simulink model "SR26_2024a"  (R2024a)
settings: Solver=FixedStepDiscrete  StartTime=0.0  StopTime=10.0  FixedStep=0.01  RelTol=1e-3  EnableMultiTasking=on
PreLoadFcn:
  | try, model_open; catch, disp('Error occurred while executing model pre-load callback: model_open.m'); disp('Please assure that the MATLAB working directory is set to the model directory before opening.'); end
InitFcn:
  | try, model_open; catch, end
values from neighbouring files (symbols this model uses):
  dt = 10.0    [SR26.sldd]
undefined symbols (not defined in the file or in its folder): GCM, raptor_get_safe_string, raptor_xcp_function
libraries: Raptor_lib x42, Utilities x6, simulink x5, IO x5, APPS_BSPC x4, Cooling x3, StateMachine x2, TorqueCommand x2, ATCC x2, BrakePressure x2, ThrottlePosition x2, Brakes x1
(part 2 of 2)

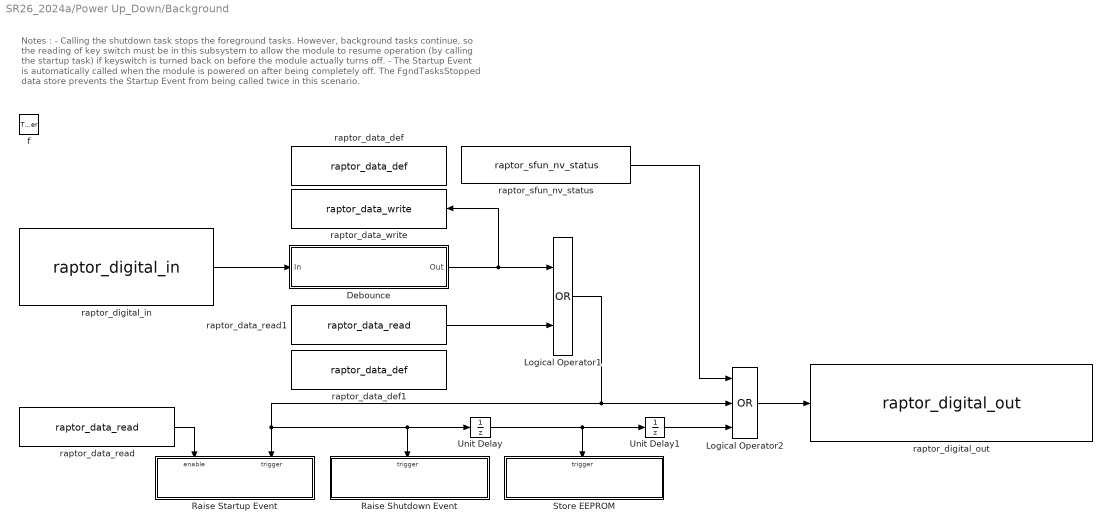
== system SR26_2024a/Power Up_Down/Background ==
  note: Notes :
      | - Calling the shutdown task stops the foreground tasks. However, background tasks continue, so the reading of key switch must be in this subsystem to allow the module
      | to resume operation (by calling the startup task) if keyswitch is turned back on before the module actually turns off.
      | - The Startup Event is automatically called when the module is powered on after being completely off. The FgndTasksStopped data store prevents the Startup Event from being called twice in this scenario.
  f : TriggerPort  TriggerType=function-call  VariantControl=Variant  ZeroCross=off
  Debounce : Subsystem
  Logical Operator1 : Logic  Operator=OR  OutDataTypeStr=boolean
  Logical Operator2 : Logic  Operator=OR  Inputs=3  OutDataTypeStr=boolean
  Raise Shutdown Event : Subsystem  TreatAsAtomicUnit=on
  Raise Startup Event : Subsystem  TreatAsAtomicUnit=on
  Store EEPROM : Subsystem  TreatAsAtomicUnit=on
  Unit Delay : UnitDelay  SampleTime=-1  HasFrameUpgradeWarning=on
  Unit Delay1 : UnitDelay  SampleTime=-1  HasFrameUpgradeWarning=on
  raptor_data_def : Raptor_lib/Data Storage/raptor_data_def  dataName='KeySw_Bgnd'  initValue=0  dataType=boolean  storage=Volatile (RAM)  calVisible=on  calType=Measurement  calDispType=Number  calEnum={'False', 'True'}  calGain=1.0  calOffset=0  calMin=-Inf  calMax=Inf  calFormat='-1'  calUnit='Bool'  calHelp='Key switch reading from background task'  calAccess=1  calFunction=group  calDispHeaders=off  calColHeaders={'Col1' 'Col2' 'Col3'}  calRowHeaders={'Row1' 'Row2' 'Row3'}
      settings: SourceProductName=Raptor
  raptor_data_def1 : Raptor_lib/Data Storage/raptor_data_def  dataName='KeepModuleOn'  initValue=0  dataType=boolean  storage=Volatile (RAM)  calVisible=on  calType=Measurement  calDispType=Number  calEnum={'False', 'True'}  calGain=1.0  calOffset=0  calMin=-Inf  calMax=Inf  calFormat='-1'  calUnit='Bool'  calHelp='Boolean indicating module to be kept on'  calAccess=1  calFunction=group  calDispHeaders=off  calColHeaders={'Col1' 'Col2' 'Col3'}  calRowHeaders={'Row1' 'Row2' 'Row3'}
      settings: SourceProductName=Raptor
  raptor_data_read : Raptor_lib/Data Storage/raptor_data_read  dataName='FgndTasksStopped'  dataShape=Scalar  idxSource=Input  idxRow=1  idxCol=1
      settings: SourceProductName=Raptor
  raptor_data_read1 : Raptor_lib/Data Storage/raptor_data_read  dataName='KeepModuleOn'  dataShape=Scalar  idxSource=Input  idxRow=1  idxCol=1
      settings: SourceProductName=Raptor
  raptor_data_write : Raptor_lib/Data Storage/raptor_data_write  dataName='KeySw_Bgnd'  dataShape=Scalar  idxSource=Input Port  idxRow=1  idxCol=1
      settings: SourceProductName=Raptor
  raptor_digital_in : Raptor_lib/Input & Output/raptor_digital_in  resourceValues=WAKE_INPUT1|INPUT33|INPUT34|INPUT35|INPUT36|INPUT37|INPUT38|INPUT39|INPUT40|(None)  resource=WAKE_INPUT1  pullUDValues=2.9k PD  pullUD=2.9k PD  upperThres=1.980  lowerThres=1.320
      settings: SourceProductName=Raptor
  raptor_digital_out : Raptor_lib/Input & Output/raptor_digital_out  resourceValues=OUTPUT9|OUTPUT21|OUTPUT22|OUTPUT23|OUTPUT24|(None)|OUTPUT1|OUTPUT2|OUTPUT3|OUTPUT4|OUTPUT5|OUTPUT6|OUTPUT7|OUTPUT8|OUTPUT10|OUTPUT11|OUTPUT25|OUTPUT26|OUTPUT27|OUTPUT28|OUTPUT29|OUTPUT30|OUTPUT31|OUTPUT32|OUTPUT33|OUTPUT34|OUTPUT35|OUTPUT36|OUTPUT37|OUTPUT38|OUTPUT39|OUTPUT40|OUTPUT41|OUTPUT42|OUTPUT43|OUTPUT44|OUTPUT45|OUTPUT46|OUTPUT47|OUTPUT48|POWER_HOLD  resource=POWER_HOLD  driverTypeValues=(None)  driverType=(None)
      settings: SourceProductName=Raptor
  raptor_sfun_nv_status : Raptor_lib/Data Storage/raptor_sfun_nv_status  showStatus=Store In Progess
      settings: SourceProductName=Raptor
  wires:
  raptor_data_read/1 -> Raise Startup Event/Enable
  raptor_digital_in/1 -> Debounce/1(In)
  Logical Operator2/1 -> raptor_digital_out/1
  Unit Delay/1 -> Store EEPROM/Trigger, Unit Delay1/1
  Logical Operator1/1 -> Logical Operator2/2, Raise Startup Event/Trigger, Raise Shutdown Event/Trigger, Unit Delay/1
  Unit Delay1/1 -> Logical Operator2/3
  raptor_sfun_nv_status/1 -> Logical Operator2/1
  raptor_data_read1/1 -> Logical Operator1/2
  Debounce/1(Out) -> raptor_data_write/1, Logical Operator1/1

== system SR26_2024a/Foreground/Controls Algorithm/APPS_BSPC ==
  IN_Inputs_Bus : Inport
  function : TriggerPort  TriggerType=function-call  VariantControl=(inherit)
  APPS : APPS_BSPC/APPS  SystemSampleTime=-1  VariantActivationTime=update diagram  EmptyChoice=off  PassThrough=off  PassThroughVariantControl=(default)  EmptyChoiceVariantControl=(default)  AllowFlexibleInterface=on  Latency=0  AutoFrameSizeCalculation=off
  BSPC : APPS_BSPC/BSPC  SystemSampleTime=-1  VariantActivationTime=update diagram  EmptyChoice=off  PassThrough=off  PassThroughVariantControl=(default)  EmptyChoiceVariantControl=(default)  AllowFlexibleInterface=on  Latency=0  AutoFrameSizeCalculation=off
  BSPCReset : APPS_BSPC/BSPCReset  SystemSampleTime=-1  VariantActivationTime=update diagram  EmptyChoice=off  PassThrough=off  PassThroughVariantControl=(default)  EmptyChoiceVariantControl=(default)  AllowFlexibleInterface=on  Latency=0  AutoFrameSizeCalculation=off
  Bus Selector : BusSelector  OutputSignals=IN_ThrottlePosition_Bus.IN_ThrottlePosition1_pct,IN_ThrottlePosition_Bus.IN_ThrottlePosition2_pct,IN_BrakePressure_Bus.IN_BrakePressureF_psi,IN_BrakePressure_Bus.IN_BrakePressureR_psi
  ThrottleSignal : APPS_BSPC/ThrottleSignal  SystemSampleTime=-1  VariantActivationTime=update diagram  EmptyChoice=off  PassThrough=off  PassThroughVariantControl=(default)  EmptyChoiceVariantControl=(default)  AllowFlexibleInterface=on  Latency=0  AutoFrameSizeCalculation=off
  CTRL_ThrottlePosition_pct : Outport
  wires:
  IN_Inputs_Bus/1 -> Bus Selector/1
  ThrottleSignal/1 -> CTRL_ThrottlePosition_pct/1
  Bus Selector/1 -> BSPC/1, BSPCReset/1, ThrottleSignal/1, APPS/1  "<IN_ThrottlePosition1_pct>"
  Bus Selector/2 -> BSPC/2, BSPCReset/2, ThrottleSignal/2, APPS/2  "<IN_ThrottlePosition2_pct>"
  Bus Selector/3 -> BSPC/3  "<IN_BrakePressureF_psi>"
  Bus Selector/4 -> BSPC/4  "<IN_BrakePressureR_psi>"

== system SR26_2024a/Foreground/Controls Algorithm/BrakeLight ==
  IN_Inputs_Bus : Inport
  function : TriggerPort  TriggerType=function-call  VariantControl=(inherit)
  BrakeLight : Brakes/BrakeLight  SystemSampleTime=-1  VariantActivationTime=update diagram  EmptyChoice=off  PassThrough=off  PassThroughVariantControl=(default)  EmptyChoiceVariantControl=(default)  AllowFlexibleInterface=on  Latency=0  AutoFrameSizeCalculation=off
  Bus Selector : BusSelector  OutputSignals=IN_BrakePressure_Bus.IN_BrakePressureF_psi,IN_BrakePressure_Bus.IN_BrakePressureR_psi
  CTRL_BrakeLight_bool : Outport
  wires:
  IN_Inputs_Bus/1 -> Bus Selector/1
  Bus Selector/1 -> BrakeLight/1  "<IN_BrakePressureF_psi>"
  Bus Selector/2 -> BrakeLight/2  "<IN_BrakePressureR_psi>"
  BrakeLight/1 -> CTRL_BrakeLight_bool/1

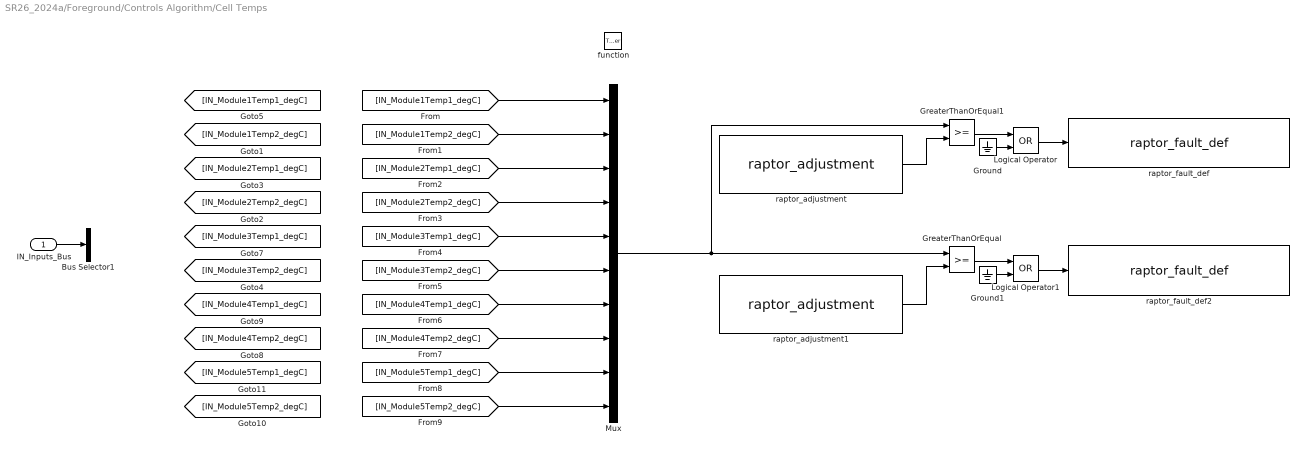
== system SR26_2024a/Foreground/Controls Algorithm/Cell Temps ==
  IN_Inputs_Bus : Inport
  function : TriggerPort  TriggerType=function-call  VariantControl=(inherit)
  Bus Selector1 : BusSelector  OutputSignals=IO_DigitalInputs_Bus.IO_CoolSwitch_bool
  GreaterThanOrEqual : RelationalOperator  OutDataTypeStr=boolean  RndMeth=Simplest  InputSameDT=off
  GreaterThanOrEqual1 : RelationalOperator  OutDataTypeStr=boolean  RndMeth=Simplest  InputSameDT=off
  Ground : Ground
  Ground1 : Ground
  Logical Operator : Logic  Operator=OR  AllPortsSameDT=off  OutDataTypeStr=boolean
  Logical Operator1 : Logic  Operator=OR  AllPortsSameDT=off  OutDataTypeStr=boolean
  Mux : Mux  Inputs=10
  raptor_adjustment : Raptor_lib/Data Storage/raptor_adjustment  paramName='CTRL_ModuleUnderThresh_degC'  nameSource=Parameter  initValue=-10  dataType=double  storage=Calibration  calDispType=Number  calEnum={'False', 'True'}  calGain=1.0  calOffset=0.0  calMax=inf  calMin=-inf  calFormat='-1'  calUnit=''  calHelp=''  calAccess=1  calFunction=raptor_xcp_function(gcb)  calDispHeaders=off  calColHeaders={'Col1' 'Col2' 'Col3'}  calRowHeaders={'Row1' 'Row2' 'Row3'}
      settings: SourceProductName=Raptor
  raptor_adjustment1 : Raptor_lib/Data Storage/raptor_adjustment  paramName='CTRL_ModuleOverTempThresh_degC'  nameSource=Parameter  initValue=55  dataType=double  storage=Calibration  calDispType=Number  calEnum={'False', 'True'}  calGain=1.0  calOffset=0.0  calMax=inf  calMin=-inf  calFormat='-1'  calUnit=''  calHelp=''  calAccess=1  calFunction=raptor_xcp_function(gcb)  calDispHeaders=off  calColHeaders={'Col1' 'Col2' 'Col3'}  calRowHeaders={'Row1' 'Row2' 'Row3'}
      settings: SourceProductName=Raptor
  raptor_fault_def : Raptor_lib/Faults/raptor_fault_def  faultName='CTRL_ModuleUnderTempFault'  persist=off  sticky=off  emisRelated=off  permanent=off  singleTrip=off  clearMethod=Standard  xLimit=25  yLimit=50  calEnable=on  addDisable=off  calAccess=1  calFunction='System | FaultManager'
      settings: SourceProductName=Raptor
  raptor_fault_def2 : Raptor_lib/Faults/raptor_fault_def  faultName='CTRL_ModuleOverTempTempFault'  persist=off  sticky=off  emisRelated=off  permanent=off  singleTrip=off  clearMethod=Standard  xLimit=25  yLimit=50  calEnable=on  addDisable=off  calAccess=1  calFunction='System | FaultManager'
      settings: SourceProductName=Raptor
  wires:
  IN_Inputs_Bus/1 -> Bus Selector1/1
  [IN_Module1Temp1_degC] -> Mux/1
  [IN_Module1Temp2_degC] -> Mux/2
  [IN_Module2Temp1_degC] -> Mux/3
  [IN_Module2Temp2_degC] -> Mux/4
  [IN_Module3Temp1_degC] -> Mux/5
  [IN_Module3Temp2_degC] -> Mux/6
  [IN_Module4Temp1_degC] -> Mux/7
  [IN_Module4Temp2_degC] -> Mux/8
  [IN_Module5Temp1_degC] -> Mux/9
  [IN_Module5Temp2_degC] -> Mux/10
  Mux/1 -> GreaterThanOrEqual1/1, GreaterThanOrEqual/1
  raptor_adjustment/1 -> GreaterThanOrEqual1/2
  raptor_adjustment1/1 -> GreaterThanOrEqual/2
  GreaterThanOrEqual1/1 -> Logical Operator/1
  Ground/1 -> Logical Operator/2
  Ground1/1 -> Logical Operator1/2
  GreaterThanOrEqual/1 -> Logical Operator1/1
  Logical Operator/1 -> raptor_fault_def/1
  Logical Operator1/1 -> raptor_fault_def2/1

== system SR26_2024a/Foreground/Controls Algorithm/ClearAllFaults ==
  function : TriggerPort  TriggerType=function-call  VariantControl=(inherit)
  raptor_fault_clear : Raptor_lib/Faults/raptor_fault_clear  faultSource=All  faultName='myFault'
      settings: SourceProductName=Raptor

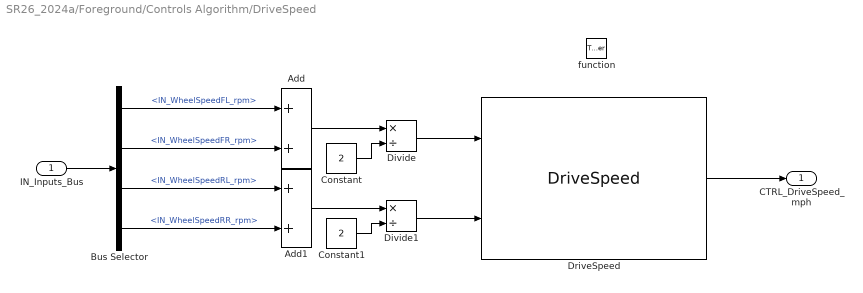
== system SR26_2024a/Foreground/Controls Algorithm/DriveSpeed ==
  IN_Inputs_Bus : Inport
  function : TriggerPort  TriggerType=function-call  VariantControl=(inherit)
  Add : Sum
  Add1 : Sum
  Bus Selector : BusSelector  OutputSignals=IN_CAN1_ATCCF_Bus.IN_WheelSpeedFL_rpm,IN_CAN1_ATCCF_Bus.IN_WheelSpeedFR_rpm,IN_CAN1_ATCCR_Bus.IN_WheelSpeedRL_rpm,IN_CAN1_ATCCR_Bus.IN_WheelSpeedRR_rpm
  Constant : Constant  Value=2
  Constant1 : Constant  Value=2
  Divide : Product  Inputs=*/
  Divide1 : Product  Inputs=*/
  DriveSpeed : DriveSpeed/DriveSpeed  SystemSampleTime=-1  VariantActivationTime=update diagram  EmptyChoice=off  PassThrough=off  PassThroughVariantControl=(default)  EmptyChoiceVariantControl=(default)  AllowFlexibleInterface=on  Latency=0  AutoFrameSizeCalculation=off
  CTRL_DriveSpeed_mph : Outport
  wires:
  IN_Inputs_Bus/1 -> Bus Selector/1
  DriveSpeed/1 -> CTRL_DriveSpeed_mph/1
  Bus Selector/1 -> Add/1  "<IN_WheelSpeedFL_rpm>"
  Bus Selector/2 -> Add/2  "<IN_WheelSpeedFR_rpm>"
  Add/1 -> Divide/1
  Constant/1 -> Divide/2
  Constant1/1 -> Divide1/2
  Add1/1 -> Divide1/1
  Bus Selector/4 -> Add1/2  "<IN_WheelSpeedRR_rpm>"
  Bus Selector/3 -> Add1/1  "<IN_WheelSpeedRL_rpm>"
  Divide/1 -> DriveSpeed/1
  Divide1/1 -> DriveSpeed/2

== system SR26_2024a/Foreground/Controls Algorithm/RTMSound ==
  CTRL_VehicleState_en : Inport
  function : TriggerPort  TriggerType=function-call  VariantControl=(inherit)
  RTMSound : StateMachine/RTMSound  SystemSampleTime=-1  VariantActivationTime=update diagram  EmptyChoice=off  PassThrough=off  PassThroughVariantControl=(default)  EmptyChoiceVariantControl=(default)  AllowFlexibleInterface=on  Latency=0  AutoFrameSizeCalculation=off
  CTRL_RTMSound_bool : Outport
  wires:
  RTMSound/1 -> CTRL_RTMSound_bool/1
  CTRL_VehicleState_en/1 -> RTMSound/1

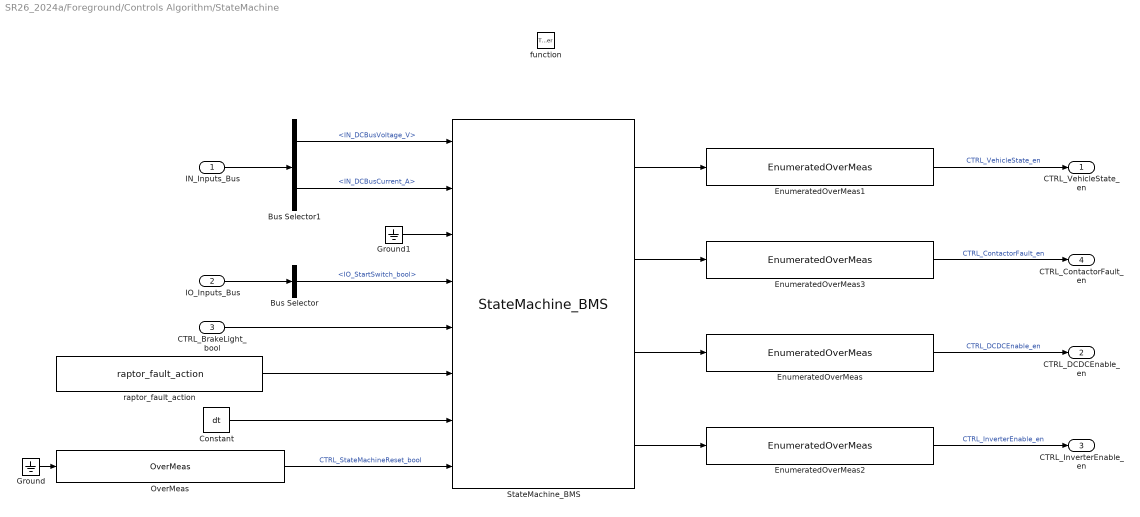
== system SR26_2024a/Foreground/Controls Algorithm/StateMachine ==
  IN_Inputs_Bus : Inport
  IO_Inputs_Bus : Inport  Port=2
  CTRL_BrakeLight_bool : Inport  Port=3
  function : TriggerPort  TriggerType=function-call  VariantControl=(inherit)
  Bus Selector : BusSelector  OutputSignals=IO_DigitalInputs_Bus.IO_StartSwitch_bool
  Bus Selector1 : BusSelector  OutputSignals=IN_CAN1_PM100DX_Bus.IN_DCBusVoltage_V,IN_CAN1_PM100DX_Bus.IN_DCBusCurrent_A
  Constant : Constant  Value=dt  OutDataTypeStr=uint32
  EnumeratedOverMeas : Utilities/EnumeratedOverMeas  sigName='CTRL_DCDCEnable_en'  enumName='DCDCEnable'
  EnumeratedOverMeas1 : Utilities/EnumeratedOverMeas  sigName='CTRL_VehicleState_en'  enumName='VehicleState'
  EnumeratedOverMeas2 : Utilities/EnumeratedOverMeas  sigName='CTRL_InverterEnable_en'  enumName='InverterEnable'
  EnumeratedOverMeas3 : Utilities/EnumeratedOverMeas  sigName='CTRL_ContactorFault_en'  enumName='ContactorFault'
  Ground : Ground
  Ground1 : Ground
  OverMeas : Utilities/OverMeas  sigName='CTRL_StateMachineReset_bool'  minimum=0  maximum=1
  StateMachine_BMS : StateMachine/StateMachine_BMS  SystemSampleTime=-1  VariantActivationTime=update diagram  EmptyChoice=off  PassThrough=off  PassThroughVariantControl=(default)  EmptyChoiceVariantControl=(default)  AllowFlexibleInterface=on  Latency=0  AutoFrameSizeCalculation=off
  raptor_fault_action : Raptor_lib/Faults/raptor_fault_action  actionName='myFaultAction'  calVisible=off  calAccess=1  calFunction='System | FaultManager | FaultAction'
      settings: SourceProductName=Raptor
  CTRL_VehicleState_en : Outport
  CTRL_DCDCEnable_en : Outport  Port=2
  CTRL_InverterEnable_en : Outport  Port=3
  CTRL_ContactorFault_en : Outport  Port=4
  wires:
  IO_Inputs_Bus/1 -> Bus Selector/1
  Bus Selector/1 -> StateMachine_BMS/4  "<IO_StartSwitch_bool>"
  IN_Inputs_Bus/1 -> Bus Selector1/1
  Bus Selector1/1 -> StateMachine_BMS/1  "<IN_DCBusVoltage_V>"
  Ground/1 -> OverMeas/1
  CTRL_BrakeLight_bool/1 -> StateMachine_BMS/5
  raptor_fault_action/1 -> StateMachine_BMS/6
  Constant/1 -> StateMachine_BMS/7
  OverMeas/1 -> StateMachine_BMS/8  "CTRL_StateMachineReset_bool"
  StateMachine_BMS/3 -> EnumeratedOverMeas/1
  StateMachine_BMS/1 -> EnumeratedOverMeas1/1
  StateMachine_BMS/4 -> EnumeratedOverMeas2/1
  EnumeratedOverMeas/1 -> CTRL_DCDCEnable_en/1  "CTRL_DCDCEnable_en"
  EnumeratedOverMeas2/1 -> CTRL_InverterEnable_en/1  "CTRL_InverterEnable_en"
  EnumeratedOverMeas1/1 -> CTRL_VehicleState_en/1  "CTRL_VehicleState_en"
  StateMachine_BMS/2 -> EnumeratedOverMeas3/1
  EnumeratedOverMeas3/1 -> CTRL_ContactorFault_en/1  "CTRL_ContactorFault_en"
  Ground1/1 -> StateMachine_BMS/3
  Bus Selector1/2 -> StateMachine_BMS/2  "<IN_DCBusCurrent_A>"

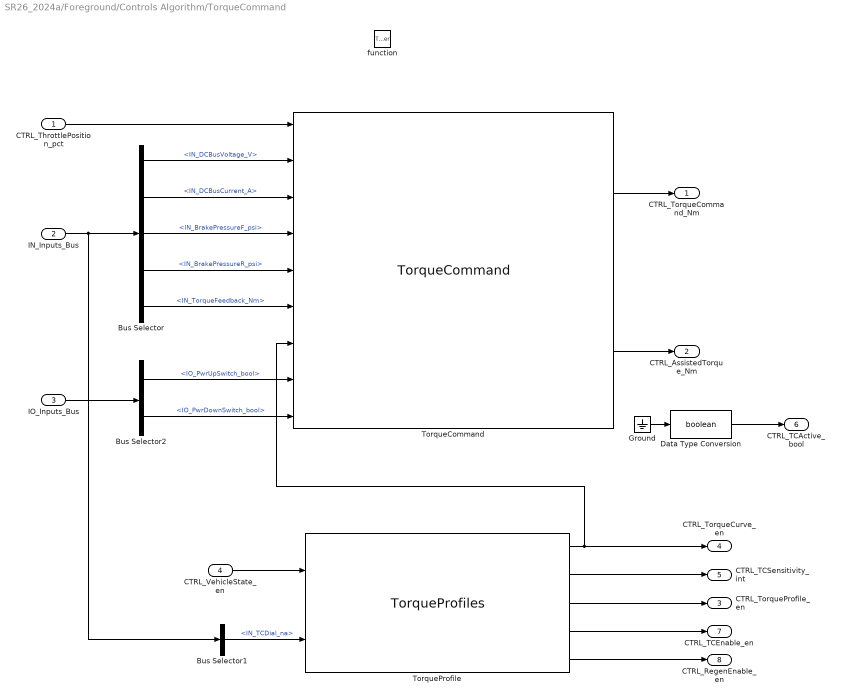
== system SR26_2024a/Foreground/Controls Algorithm/TorqueCommand ==
  CTRL_ThrottlePosition_pct : Inport
  IN_Inputs_Bus : Inport  Port=2
  IO_Inputs_Bus : Inport  Port=3
  CTRL_VehicleState_en : Inport  Port=4
  function : TriggerPort  TriggerType=function-call  VariantControl=(inherit)
  Bus Selector : BusSelector  OutputSignals=IN_CAN1_PM100DX_Bus.IN_DCBusVoltage_V,IN_CAN1_PM100DX_Bus.IN_DCBusCurrent_A,IN_BrakePressure_Bus.IN_BrakePressureF_psi,IN_BrakePressure_Bus.IN_BrakePressureR_psi,IN_CAN1_PM100DX_Bus.IN_TorqueFeedback_Nm
  Bus Selector1 : BusSelector  OutputSignals=IN_TCDial_na
  Bus Selector2 : BusSelector  OutputSignals=IO_DigitalInputs_Bus.IO_PwrUpSwitch_bool,IO_DigitalInputs_Bus.IO_PwrDownSwitch_bool
  Data Type Conversion : DataTypeConversion  OutDataTypeStr=boolean  SaturateOnIntegerOverflow=off  RndMeth=Floor
  Ground : Ground
  TorqueCommand : TorqueCommand/TorqueCommand  SystemSampleTime=-1  VariantActivationTime=update diagram  EmptyChoice=off  PassThrough=off  PassThroughVariantControl=(default)  EmptyChoiceVariantControl=(default)  AllowFlexibleInterface=on  Latency=0  AutoFrameSizeCalculation=off
  TorqueProfile : TorqueCommand/TorqueProfiles  SystemSampleTime=-1  VariantActivationTime=update diagram  EmptyChoice=off  PassThrough=off  PassThroughVariantControl=(default)  EmptyChoiceVariantControl=(default)  AllowFlexibleInterface=on  Latency=0  AutoFrameSizeCalculation=off
  CTRL_TorqueCommand_Nm : Outport  VectorParamsAs1DForOutWhenUnconnected=off
  CTRL_AssistedTorque_Nm : Outport  Port=2  VectorParamsAs1DForOutWhenUnconnected=off
  CTRL_TorqueProfile_en : Outport  Port=3  VectorParamsAs1DForOutWhenUnconnected=off
  CTRL_TorqueCurve_en : Outport  Port=4  VectorParamsAs1DForOutWhenUnconnected=off
  CTRL_TCSensitivity_int : Outport  Port=5  VectorParamsAs1DForOutWhenUnconnected=off
  CTRL_TCActive_bool : Outport  Port=6  VectorParamsAs1DForOutWhenUnconnected=off
  CTRL_TCEnable_en : Outport  Port=7  VectorParamsAs1DForOutWhenUnconnected=off
  CTRL_RegenEnable_en : Outport  Port=8  VectorParamsAs1DForOutWhenUnconnected=off
  wires:
  CTRL_ThrottlePosition_pct/1 -> TorqueCommand/1
  TorqueCommand/1 -> CTRL_TorqueCommand_Nm/1
  IN_Inputs_Bus/1 -> Bus Selector1/1, Bus Selector/1
  TorqueProfile/1 -> TorqueCommand/7, CTRL_TorqueCurve_en/1
  IO_Inputs_Bus/1 -> Bus Selector2/1
  Bus Selector1/1 -> TorqueProfile/2  "<IN_TCDial_na>"
  TorqueProfile/2 -> CTRL_TCSensitivity_int/1
  TorqueProfile/3 -> CTRL_TorqueProfile_en/1
  CTRL_VehicleState_en/1 -> TorqueProfile/1
  Bus Selector2/1 -> TorqueCommand/8  "<IO_PwrUpSwitch_bool>"
  Bus Selector2/2 -> TorqueCommand/9  "<IO_PwrDownSwitch_bool>"
  Bus Selector/3 -> TorqueCommand/4  "<IN_BrakePressureF_psi>"
  Bus Selector/4 -> TorqueCommand/5  "<IN_BrakePressureR_psi>"
  TorqueCommand/2 -> CTRL_AssistedTorque_Nm/1
  Bus Selector/5 -> TorqueCommand/6  "<IN_TorqueFeedback_Nm>"
  Bus Selector/1 -> TorqueCommand/2  "<IN_DCBusVoltage_V>"
  Bus Selector/2 -> TorqueCommand/3  "<IN_DCBusCurrent_A>"
  TorqueProfile/4 -> CTRL_TCEnable_en/1
  TorqueProfile/5 -> CTRL_RegenEnable_en/1
  Ground/1 -> Data Type Conversion/1
  Data Type Conversion/1 -> CTRL_TCActive_bool/1

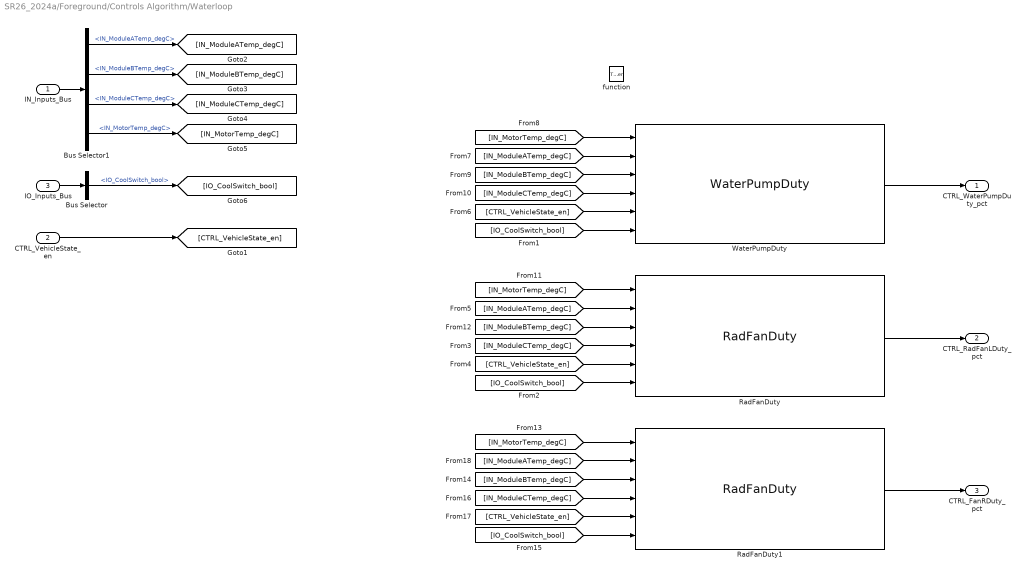
== system SR26_2024a/Foreground/Controls Algorithm/Waterloop ==
  IN_Inputs_Bus : Inport
  CTRL_VehicleState_en : Inport  Port=2
  IO_Inputs_Bus : Inport  Port=3
  function : TriggerPort  TriggerType=function-call  VariantControl=(inherit)
  Bus Selector : BusSelector  OutputSignals=IO_DigitalInputs_Bus.IO_CoolSwitch_bool
  Bus Selector1 : BusSelector  OutputSignals=IN_CAN1_PM100DX_Bus.IN_ModuleATemp_degC,IN_CAN1_PM100DX_Bus.IN_ModuleBTemp_degC,IN_CAN1_PM100DX_Bus.IN_ModuleCTemp_degC,IN_CAN1_PM100DX_Bus.IN_MotorTemp_degC
  RadFanDuty : Cooling/RadFanDuty  pos='L'
  RadFanDuty1 : Cooling/RadFanDuty  pos='R'
  WaterPumpDuty : Cooling/WaterPumpDuty
  CTRL_WaterPumpDuty_pct : Outport
  CTRL_RadFanLDuty_pct : Outport  Port=2
  CTRL_FanRDuty_pct : Outport  Port=3
  wires:
  RadFanDuty/1 -> CTRL_RadFanLDuty_pct/1
  WaterPumpDuty/1 -> CTRL_WaterPumpDuty_pct/1
  IO_Inputs_Bus/1 -> Bus Selector/1
  Bus Selector/1 -> [IO_CoolSwitch_bool]  "<IO_CoolSwitch_bool>"
  CTRL_VehicleState_en/1 -> [CTRL_VehicleState_en]
  [CTRL_VehicleState_en] -> WaterPumpDuty/5
  [IO_CoolSwitch_bool] -> WaterPumpDuty/6
  RadFanDuty1/1 -> CTRL_FanRDuty_pct/1
  IN_Inputs_Bus/1 -> Bus Selector1/1
  [IN_ModuleATemp_degC] -> WaterPumpDuty/2
  [IN_MotorTemp_degC] -> WaterPumpDuty/1
  [IN_ModuleBTemp_degC] -> WaterPumpDuty/3
  [IN_ModuleCTemp_degC] -> WaterPumpDuty/4
  [IN_ModuleCTemp_degC] -> RadFanDuty/4
  [IN_ModuleBTemp_degC] -> RadFanDuty/3
  [IN_MotorTemp_degC] -> RadFanDuty/1
  [IN_ModuleATemp_degC] -> RadFanDuty/2
  [IO_CoolSwitch_bool] -> RadFanDuty/6
  [CTRL_VehicleState_en] -> RadFanDuty/5
  [CTRL_VehicleState_en] -> RadFanDuty1/5
  [IO_CoolSwitch_bool] -> RadFanDuty1/6
  [IN_ModuleATemp_degC] -> RadFanDuty1/2
  [IN_MotorTemp_degC] -> RadFanDuty1/1
  [IN_ModuleBTemp_degC] -> RadFanDuty1/3
  [IN_ModuleCTemp_degC] -> RadFanDuty1/4
  Bus Selector1/1 -> [IN_ModuleATemp_degC]  "<IN_ModuleATemp_degC>"
  Bus Selector1/2 -> [IN_ModuleBTemp_degC]  "<IN_ModuleBTemp_degC>"
  Bus Selector1/3 -> [IN_ModuleCTemp_degC]  "<IN_ModuleCTemp_degC>"
  Bus Selector1/4 -> [IN_MotorTemp_degC]  "<IN_MotorTemp_degC>"

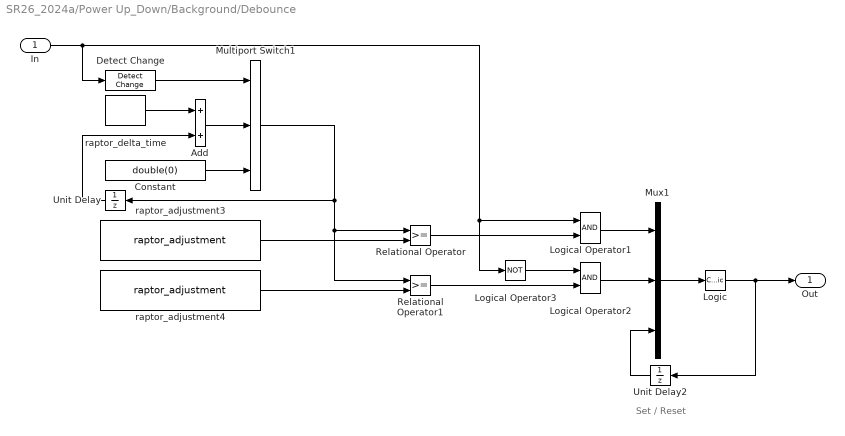
== system SR26_2024a/Power Up_Down/Background/Debounce ==
  note: Set / Reset
  In : Inport
  Add : Sum
  Constant : Constant  Value=double(0)
  Detect Change : simulink/Logic and Bit Operations/Detect Change  vinit=0  OutDataTypeStr=boolean
  Logic : CombinatorialLogic  TruthTable=[0;1;0;0;1;1;0;0]
  Logical Operator1 : Logic  AllPortsSameDT=off  OutDataTypeStr=boolean
  Logical Operator2 : Logic  AllPortsSameDT=off  OutDataTypeStr=boolean
  Logical Operator3 : Logic  Operator=NOT  Inputs=1  AllPortsSameDT=off  OutDataTypeStr=boolean
  Multiport Switch1 : MultiPortSwitch  DataPortOrder=Zero-based contiguous  Inputs=2  zeroidx=on  SaturateOnIntegerOverflow=off  InputSameDT=off
  Mux1 : Mux  Inputs=3
  Relational Operator : RelationalOperator  OutDataTypeStr=boolean  InputSameDT=off
  Relational Operator1 : RelationalOperator  OutDataTypeStr=boolean  InputSameDT=off
  Unit Delay : UnitDelay  SampleTime=-1  HasFrameUpgradeWarning=on
  Unit Delay2 : UnitDelay  InitialCondition=1  SampleTime=-1  HasFrameUpgradeWarning=on
  raptor_adjustment3 : Raptor_lib/Data Storage/raptor_adjustment  paramName='KeySwHiTimeThr'  nameSource=Parameter  initValue=0.2  dataType=double  storage=Calibration  calDispType=Number  calEnum={'Active Low', 'Active High'}  calGain=1  calOffset=0  calMax=inf  calMin=-inf  calFormat='-1'  calUnit='sec'  calHelp='State high time threshold'  calAccess=1  calFunction=group  calDispHeaders=off  calColHeaders={'Col1' 'Col2' 'Col3'}  calRowHeaders={'Row1' 'Row2' 'Row3'}
      settings: SourceProductName=Raptor
  raptor_adjustment4 : Raptor_lib/Data Storage/raptor_adjustment  paramName='KeySwLoTimeThr'  nameSource=Parameter  initValue=0.2  dataType=double  storage=Calibration  calDispType=Number  calEnum={'Active Low', 'Active High'}  calGain=1  calOffset=0  calMax=inf  calMin=-inf  calFormat='-1'  calUnit='sec'  calHelp='State low time threshold'  calAccess=1  calFunction=group  calDispHeaders=off  calColHeaders={'Col1' 'Col2' 'Col3'}  calRowHeaders={'Row1' 'Row2' 'Row3'}
      settings: SourceProductName=Raptor
  raptor_delta_time : Raptor_lib/Triggers/raptor_delta_time  unit=seconds
      settings: SourceProductName=Raptor
  Out : Outport  VectorParamsAs1DForOutWhenUnconnected=off
  wires:
  Detect Change/1 -> Multiport Switch1/1
  Logical Operator3/1 -> Logical Operator2/1
  Relational Operator/1 -> Logical Operator1/2
  Logical Operator2/1 -> Mux1/2
  Logical Operator1/1 -> Mux1/1
  Mux1/1 -> Logic/1
  Unit Delay2/1 -> Mux1/3
  In/1 -> Detect Change/1, Logical Operator1/1, Logical Operator3/1
  Multiport Switch1/1 -> Unit Delay/1, Relational Operator/1, Relational Operator1/1
  Add/1 -> Multiport Switch1/2
  Constant/1 -> Multiport Switch1/3
  Relational Operator1/1 -> Logical Operator2/2
  Logic/1 -> Unit Delay2/1, Out/1
  Unit Delay/1 -> Add/2
  raptor_delta_time/1 -> Add/1
  raptor_adjustment4/1 -> Relational Operator1/2
  raptor_adjustment3/1 -> Relational Operator/2

== system SR26_2024a/Power Up_Down/Background/Raise Shutdown Event ==
  Trigger : TriggerPort  TriggerType=falling  VariantControl=Variant
  Constant : Constant  Value=boolean(1)
  Function-Call Generator : simulink/Ports & Subsystems/Function-Call Generator  sample_time=-1  numberOfIterations=1  DisallowWideOutput=off
  raptor_data_def : Raptor_lib/Data Storage/raptor_data_def  dataName='FgndTasksStopped'  initValue=0  dataType=boolean  storage=Volatile (RAM)  calVisible=on  calType=Measurement  calDispType=Number  calEnum={'False', 'True'}  calGain=1.0  calOffset=0  calMin=-Inf  calMax=Inf  calFormat='-1'  calUnit='Bool'  calHelp='Boolean indicating foreground tasks stopped'  calAccess=1  calFunction=group  calDispHeaders=off  calColHeaders={'Col1' 'Col2' 'Col3'}  calRowHeaders={'Row1' 'Row2' 'Row3'}
      settings: SourceProductName=Raptor
  raptor_data_write : Raptor_lib/Data Storage/raptor_data_write  dataName='FgndTasksStopped'  dataShape=Scalar  idxSource=Input Port  idxRow=1  idxCol=1
      settings: SourceProductName=Raptor
  raptor_shutdown : Raptor_lib/Triggers/raptor_shutdown  null=0
      settings: SourceProductName=Raptor
  wires:
  Constant/1 -> raptor_data_write/1
  Function-Call Generator/1 -> raptor_shutdown/Trigger

== system SR26_2024a/Power Up_Down/Background/Raise Startup Event ==
  Enable : EnablePort
  Trigger : TriggerPort  VariantControl=Variant
  Function-Call Generator : simulink/Ports & Subsystems/Function-Call Generator  sample_time=-1  numberOfIterations=1  DisallowWideOutput=off
  raptor_startup : Raptor_lib/Triggers/raptor_startup  null=0
      settings: SourceProductName=Raptor
  wires:
  Function-Call Generator/1 -> raptor_startup/Trigger

== system SR26_2024a/Power Up_Down/Background/Store EEPROM ==
  Trigger : TriggerPort  TriggerType=falling  VariantControl=Variant
  Function-Call Generator : simulink/Ports & Subsystems/Function-Call Generator  sample_time=-1  numberOfIterations=1  DisallowWideOutput=off
  raptor_store_nv : Raptor_lib/Data Storage/raptor_store_nv  null=0
      settings: SourceProductName=Raptor
  wires:
  Function-Call Generator/1 -> raptor_store_nv/Trigger
